simulink model "simulacao"  (R2025a)
settings: Solver=VariableStepAuto  StartTime=0.0  StopTime=10.0  RelTol=1e-3
settings Model: Creator=luiza  LastModifiedBy=luiza

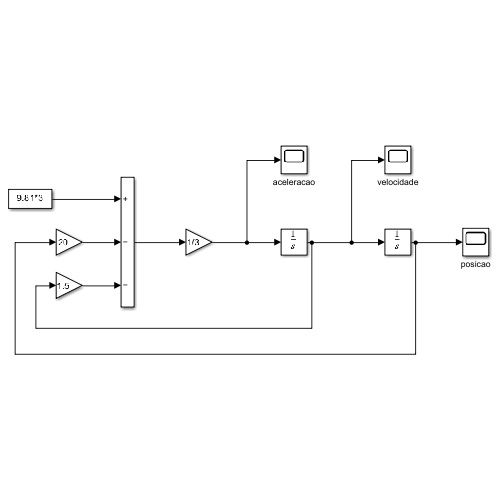
[thumbnail: Simulink's stored preview of the top-level diagram]
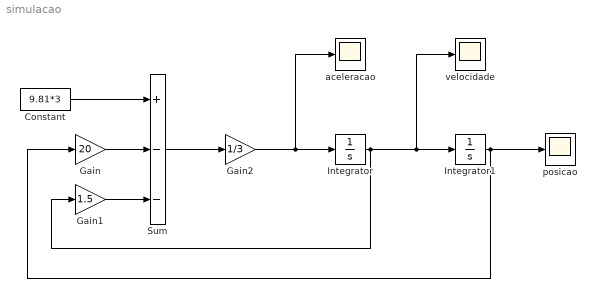
== system simulacao ==
  Constant : Constant  Value=9.81*3
  Gain : Gain  Gain=20
  Gain1 : Gain  Gain=1.5
  Gain2 : Gain  Gain=1/3
  Integrator : Integrator
  Integrator1 : Integrator
  Sum : Sum  Inputs=+--
  aceleracao : Scope
      settings: ActiveDisplayYMinimum=-9.3156704991251367  ActiveDisplayYMaximum=11.935074499902791  DataLoggingVariableName=ScopeData2
  posicao : Scope
      settings: ActiveDisplayYMinimum=-0.31868529141325491  ActiveDisplayYMaximum=2.8681676227192945
  velocidade : Scope
      settings: ActiveDisplayYMinimum=-3.0879508465482637  ActiveDisplayYMaximum=3.9042103438153126
  wires:
  Constant/1 -> Sum/1
  Gain1/1 -> Sum/3
  Gain/1 -> Sum/2
  Sum/1 -> Gain2/1
  Gain2/1 -> aceleracao/1, Integrator/1
  Integrator/1 -> Gain1/1, velocidade/1, Integrator1/1
  Integrator1/1 -> Gain/1, posicao/1
